simulink model "ddc_bpm_476_066"  (Simulink 7.8)
settings: Solver=ode45  StartTime=0.0  StopTime=2e-3  RelTol=1e-3
undefined symbols (not defined in the file): decim_factor_poly_35, dt_sim, frev_476, Fs_adc, n_ch, n_ovs, R_fofb, R_sec, R_sec_cfir, R_sec_pfir, xlipgetpartsetting
libraries: xbsIndex_r4 x1436, simulink x7
(part 3 of 12)

== system ddc_bpm_476_066/ST3 ==
  In : Inport
  Display : Display
  Sample Time : xbsIndex_r4/Sample Time  block_type=sampletime
      settings: infoedit="The Sample Time block reports the normalized sample period of its input.  A signal's normalized sample period is not equivalent to its Simulink absolute sample period.<br><br>Hardware notes: This block is implemented as a constant in hardware."
  out : xbsIndex_r4/Gateway Out  inherit_from_input=on  hdl_port=off  timing_constraint=Data Rate  locs_specified=off  LOCs={}  UseAsDAC=off  DACChannel='1'  block_type=gatewayout
      settings: infoedit="Gateway out block.  Converts Xilinx fixed-point or floating-point type inputs into ouputs of type Simulink integer, single, double, or fixed point.<br><br>Hardware notes:  In hardware these blocks become top level output ports or are discarded, depending on how they are configured."
  wires:
  out/1 -> Display/1
  Sample Time/1 -> out/1
  In/1 -> Sample Time/1

== system ddc_bpm_476_066/ST4 ==
  In : Inport
  Display : Display
  Sample Time : xbsIndex_r4/Sample Time  block_type=sampletime
      settings: infoedit="The Sample Time block reports the normalized sample period of its input.  A signal's normalized sample period is not equivalent to its Simulink absolute sample period.<br><br>Hardware notes: This block is implemented as a constant in hardware."
  out : xbsIndex_r4/Gateway Out  inherit_from_input=on  hdl_port=off  timing_constraint=Data Rate  locs_specified=off  LOCs={}  UseAsDAC=off  DACChannel='1'  block_type=gatewayout
      settings: infoedit="Gateway out block.  Converts Xilinx fixed-point or floating-point type inputs into ouputs of type Simulink integer, single, double, or fixed point.<br><br>Hardware notes:  In hardware these blocks become top level output ports or are discarded, depending on how they are configured."
  wires:
  out/1 -> Display/1
  Sample Time/1 -> out/1
  In/1 -> Sample Time/1

== system ddc_bpm_476_066/ST5 ==
  In : Inport
  Display : Display
  Sample Time : xbsIndex_r4/Sample Time  block_type=sampletime
      settings: infoedit="The Sample Time block reports the normalized sample period of its input.  A signal's normalized sample period is not equivalent to its Simulink absolute sample period.<br><br>Hardware notes: This block is implemented as a constant in hardware."
  out : xbsIndex_r4/Gateway Out  inherit_from_input=on  hdl_port=off  timing_constraint=Data Rate  locs_specified=off  LOCs={}  UseAsDAC=off  DACChannel='1'  block_type=gatewayout
      settings: infoedit="Gateway out block.  Converts Xilinx fixed-point or floating-point type inputs into ouputs of type Simulink integer, single, double, or fixed point.<br><br>Hardware notes:  In hardware these blocks become top level output ports or are discarded, depending on how they are configured."
  wires:
  out/1 -> Display/1
  Sample Time/1 -> out/1
  In/1 -> Sample Time/1

== system ddc_bpm_476_066/ST6 ==
  In : Inport
  Display : Display
  Sample Time : xbsIndex_r4/Sample Time  block_type=sampletime
      settings: infoedit="The Sample Time block reports the normalized sample period of its input.  A signal's normalized sample period is not equivalent to its Simulink absolute sample period.<br><br>Hardware notes: This block is implemented as a constant in hardware."
  out : xbsIndex_r4/Gateway Out  inherit_from_input=on  hdl_port=off  timing_constraint=Data Rate  locs_specified=off  LOCs={}  UseAsDAC=off  DACChannel='1'  block_type=gatewayout
      settings: infoedit="Gateway out block.  Converts Xilinx fixed-point or floating-point type inputs into ouputs of type Simulink integer, single, double, or fixed point.<br><br>Hardware notes:  In hardware these blocks become top level output ports or are discarded, depending on how they are configured."
  wires:
  out/1 -> Display/1
  Sample Time/1 -> out/1
  In/1 -> Sample Time/1

== system ddc_bpm_476_066/ST7 ==
  In : Inport
  Display : Display
  Sample Time : xbsIndex_r4/Sample Time  block_type=sampletime
      settings: infoedit="The Sample Time block reports the normalized sample period of its input.  A signal's normalized sample period is not equivalent to its Simulink absolute sample period.<br><br>Hardware notes: This block is implemented as a constant in hardware."
  out : xbsIndex_r4/Gateway Out  inherit_from_input=on  hdl_port=off  timing_constraint=Data Rate  locs_specified=off  LOCs={}  UseAsDAC=off  DACChannel='1'  block_type=gatewayout
      settings: infoedit="Gateway out block.  Converts Xilinx fixed-point or floating-point type inputs into ouputs of type Simulink integer, single, double, or fixed point.<br><br>Hardware notes:  In hardware these blocks become top level output ports or are discarded, depending on how they are configured."
  wires:
  out/1 -> Display/1
  Sample Time/1 -> out/1
  In/1 -> Sample Time/1

== system ddc_bpm_476_066/ST8 ==
  In : Inport
  Display : Display
  Sample Time : xbsIndex_r4/Sample Time  block_type=sampletime
      settings: infoedit="The Sample Time block reports the normalized sample period of its input.  A signal's normalized sample period is not equivalent to its Simulink absolute sample period.<br><br>Hardware notes: This block is implemented as a constant in hardware."
  X_monit1 : xbsIndex_r4/Gateway Out  inherit_from_input=on  hdl_port=off  timing_constraint=Data Rate  locs_specified=off  LOCs={}  UseAsDAC=off  DACChannel='1'  block_type=gatewayout
      settings: infoedit="Gateway out block.  Converts Xilinx fixed-point or floating-point type inputs into ouputs of type Simulink integer, single, double, or fixed point.<br><br>Hardware notes:  In hardware these blocks become top level output ports or are discarded, depending on how they are configured."
  wires:
  X_monit1/1 -> Display/1
  Sample Time/1 -> X_monit1/1
  In/1 -> Sample Time/1

== system ddc_bpm_476_066/ST9 ==
  In : Inport
  Display : Display
  Sample Time : xbsIndex_r4/Sample Time  block_type=sampletime
      settings: infoedit="The Sample Time block reports the normalized sample period of its input.  A signal's normalized sample period is not equivalent to its Simulink absolute sample period.<br><br>Hardware notes: This block is implemented as a constant in hardware."
  out : xbsIndex_r4/Gateway Out  inherit_from_input=on  hdl_port=off  timing_constraint=Data Rate  locs_specified=off  LOCs={}  UseAsDAC=off  DACChannel='1'  block_type=gatewayout
      settings: infoedit="Gateway out block.  Converts Xilinx fixed-point or floating-point type inputs into ouputs of type Simulink integer, single, double, or fixed point.<br><br>Hardware notes:  In hardware these blocks become top level output ports or are discarded, depending on how they are configured."
  wires:
  out/1 -> Display/1
  Sample Time/1 -> out/1
  In/1 -> Sample Time/1

== system ddc_bpm_476_066/TBT_amp ==
  Q_in0 : Inport
  I_in0 : Inport  Port=2
  ch_in0 : Inport  Port=3
  Q_in1 : Inport  Port=4
  I_in1 : Inport  Port=5
  ch_in1 : Inport  Port=6
  ST5 : Subsystem
  TBT_amp0 : Subsystem
  TBT_amp1 : Subsystem
  TDDM_tbt_amp_4ch : Subsystem
  Terminator{,1,3..4} (4 alike) : Terminator
  amp_out0 : Outport
  amp_out1 : Outport  Port=2
  amp_out2 : Outport  Port=3
  amp_out3 : Outport  Port=4
  wires:
  Q_in0/1 -> TBT_amp0/1(Q_in)
  I_in0/1 -> TBT_amp0/2(I_in)
  ch_in0/1 -> TBT_amp0/3(ch_in)
  Q_in1/1 -> TBT_amp1/1(Q_in)
  I_in1/1 -> TBT_amp1/2(I_in)
  ch_in1/1 -> TBT_amp1/3(ch_in)
  TBT_amp0/2(phase_out) -> Terminator/1
  TBT_amp0/3(valid_out) -> Terminator1/1
  TBT_amp1/2(phase_out) -> Terminator3/1
  TBT_amp1/3(valid_out) -> Terminator4/1
  TBT_amp0/1(amp_out) -> TDDM_tbt_amp_4ch/1(amp_in0), ST5/1(In)
  TBT_amp0/4(ch_out) -> TDDM_tbt_amp_4ch/2(ch_in0)
  TBT_amp1/1(amp_out) -> TDDM_tbt_amp_4ch/3(amp_in1)
  TBT_amp1/4(ch_out) -> TDDM_tbt_amp_4ch/4(ch_in1)
  TDDM_tbt_amp_4ch/1(amp_out0) -> amp_out0/1
  TDDM_tbt_amp_4ch/2(amp_out1) -> amp_out1/1
  TDDM_tbt_amp_4ch/3(amp_out2) -> amp_out2/1
  TDDM_tbt_amp_4ch/4(amp_out3) -> amp_out3/1

== system ddc_bpm_476_066/TDM_mix ==
  din_ch0 : Inport
  din_ch1 : Inport  Port=2
  din_ch2 : Inport  Port=3
  din_ch3 : Inport  Port=4
  Constant10 : xbsIndex_r4/Constant  const=0  gui_display_data_type=Boolean  arith_type=Boolean  n_bits=16  bin_pt=14  preci_type=Single  exp_width=8  frac_width=24  explicit_period=on  period=1/Fs_adc/n_ovs  equ=P=C  opselect=C  inp2=PCIN>>17  opr=+  inp1=P  carry=CIN  dbl_ovrd=off  block_type=constant
  Constant11 : xbsIndex_r4/Constant  const=0  gui_display_data_type=Boolean  arith_type=Boolean  n_bits=16  bin_pt=14  preci_type=Single  exp_width=8  frac_width=24  explicit_period=on  period=1/Fs_adc/n_ovs  equ=P=C  opselect=C  inp2=PCIN>>17  opr=+  inp1=P  carry=CIN  dbl_ovrd=off  block_type=constant
  ST1 : Subsystem
  ST2 : Subsystem
  ST3 : Subsystem
  ST4 : Subsystem
  ST5 : Subsystem
  ST6 : Subsystem
  TDM_mix_ch0_1 : Subsystem
  TDM_mix_ch0_2 : Subsystem
  dout0 : Outport
  ch_out0 : Outport  Port=2
  dout1 : Outport  Port=3
  ch_out1 : Outport  Port=4
  wires:
  Constant10/1 -> TDM_mix_ch0_1/1(rst), ST3/1(In)
  Constant11/1 -> ST5/1(In), TDM_mix_ch0_2/1(rst)
  TDM_mix_ch0_1/1(dout) -> dout0/1, ST1/1(In)
  din_ch0/1 -> TDM_mix_ch0_1/2(din_ch0)
  TDM_mix_ch0_1/2(ch_out) -> ch_out0/1
  din_ch1/1 -> TDM_mix_ch0_1/3(din_ch1), ST2/1(In)
  TDM_mix_ch0_2/1(dout) -> dout1/1, ST4/1(In)
  din_ch2/1 -> TDM_mix_ch0_2/2(din_ch0)
  TDM_mix_ch0_2/2(ch_out) -> ch_out1/1
  din_ch3/1 -> ST6/1(In), TDM_mix_ch0_2/3(din_ch1)

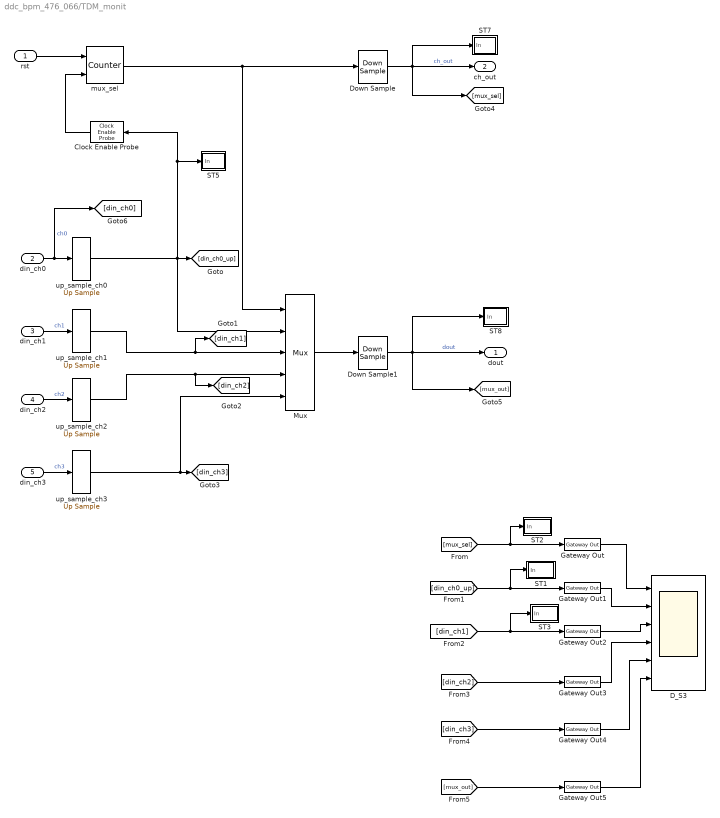
== system ddc_bpm_476_066/TDM_monit ==
  rst : Inport
  din_ch0 : Inport  Port=2
  din_ch1 : Inport  Port=3
  din_ch2 : Inport  Port=4
  din_ch3 : Inport  Port=5
  Clock Enable Probe : xbsIndex_r4/Clock Enable Probe  inherit_constraints=on  block_type=ceprobe
      settings: infoedit="Clock enable extractor.  Produces a Boolean output that mirrors the hardware clock enable associated with the input sample rate.<br><br>Hardware notes: in hardware this block costs nothing."
  D_S3 : Scope  NumInputPorts=6
      settings: TimeRange=0.0004  YMin=-1~-1.5~10~-1.5~-5~-5  YMax=1~1.5~100~1.5~5~5  MaxDataPoints=1000000  SampleInput=on
  Down Sample : xbsIndex_r4/Down Sample  sample_ratio=R_fofb*n_ovs/n_ch  sample_phase="Last Value of Frame  (most efficient)"  en=off  latency=1  dbl_ovrd=off  block_type=dsamp
  Down Sample1 : xbsIndex_r4/Down Sample  sample_ratio=R_fofb*n_ovs/n_ch  sample_phase="Last Value of Frame  (most efficient)"  en=off  latency=1  dbl_ovrd=off  block_type=dsamp
  Gateway Out{,1..5} (6 alike) : xbsIndex_r4/Gateway Out  inherit_from_input=on  hdl_port=off  timing_constraint=None  locs_specified=off  LOCs={}  UseAsDAC=off  DACChannel='1'  block_type=gatewayout
      settings: infoedit="Gateway out block.  Converts Xilinx fixed-point or floating-point type inputs into ouputs of type Simulink integer, single, double, or fixed point.<br><br>Hardware notes:  In hardware these blocks become top level output ports or are discarded, depending on how they are configured."
  Mux : xbsIndex_r4/Mux  inputs=4  en=off  latency=0  precision=Full  arith_type=Unsigned  n_bits=16  bin_pt=14  quantization=Truncate  overflow=Wrap  dbl_ovrd=off  block_type=mux
  ST1 : Subsystem
  ST2 : Subsystem
  ST3 : Subsystem
  ST5 : Subsystem
  ST7 : Subsystem
  ST8 : Subsystem
  mux_sel : xbsIndex_r4/Counter  cnt_type=Free Running  cnt_to=Inf  operation=Up  start_count=0  cnt_by_val=1  arith_type=Unsigned  n_bits=2  bin_pt=0  load_pin=off  rst=on  en=on  explicit_period=off  period=1/Fs_adc/4*1112  dbl_ovrd=off  use_behavioral_HDL=off  implementation=Fabric  block_type=counter
  up_sample_ch{0..3} (4 alike) : xbsIndex_r4/Up Sample  sample_ratio=n_ch  copy_samples=on  en=off  latency=0  dbl_ovrd=off  block_type=usamp
  dout : Outport
  ch_out : Outport  Port=2
  wires:
  Mux/1 -> Down Sample1/1
  mux_sel/1 -> Mux/1, Down Sample/1
  up_sample_ch3/1 -> Mux/5, [din_ch3]
  up_sample_ch2/1 -> Mux/4, [din_ch2]
  up_sample_ch1/1 -> Mux/3, [din_ch1]
  up_sample_ch0/1 -> Mux/2, [din_ch0_up], Clock Enable Probe/1, ST5/1(In)
  din_ch0/1 -> [din_ch0], up_sample_ch0/1  "ch0"
  din_ch1/1 -> up_sample_ch1/1  "ch1"
  Down Sample1/1 -> dout/1, [mux_out], ST8/1(In)  "dout"
  din_ch2/1 -> up_sample_ch2/1  "ch2"
  din_ch3/1 -> up_sample_ch3/1  "ch3"
  Down Sample/1 -> ch_out/1, [mux_sel], ST7/1(In)  "ch_out"
  Gateway Out/1 -> D_S3/1
  Gateway Out1/1 -> D_S3/2
  Gateway Out4/1 -> D_S3/5
  Gateway Out3/1 -> D_S3/4
  Gateway Out2/1 -> D_S3/3
  [mux_sel] -> Gateway Out/1, ST2/1(In)
  [din_ch0_up] -> Gateway Out1/1, ST1/1(In)
  [din_ch1] -> Gateway Out2/1, ST3/1(In)
  [din_ch3] -> Gateway Out4/1
  [din_ch2] -> Gateway Out3/1
  [mux_out] -> Gateway Out5/1
  Gateway Out5/1 -> D_S3/6
  Clock Enable Probe/1 -> mux_sel/2
  rst/1 -> mux_sel/1

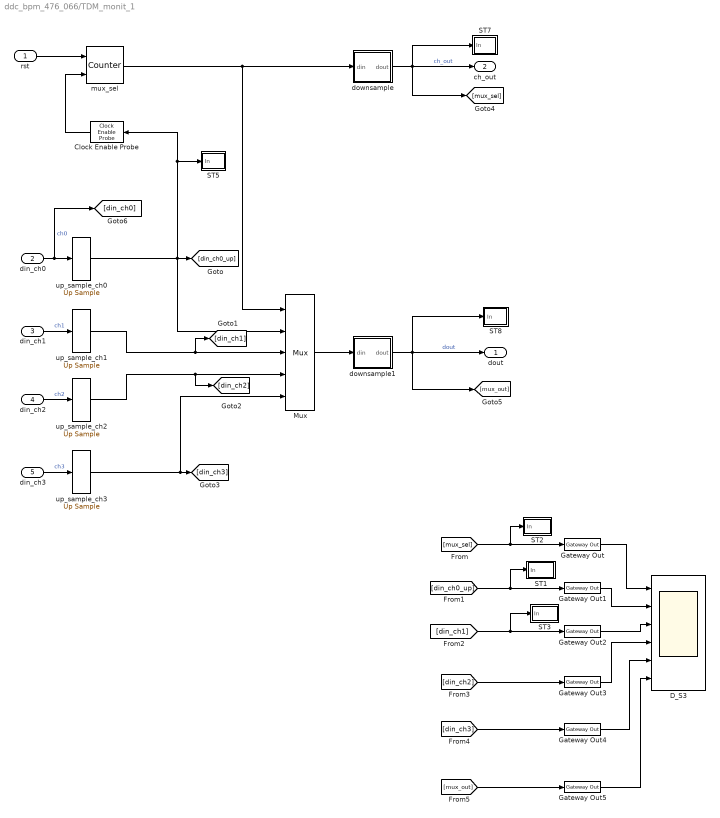
== system ddc_bpm_476_066/TDM_monit_1 ==
  rst : Inport
  din_ch0 : Inport  Port=2
  din_ch1 : Inport  Port=3
  din_ch2 : Inport  Port=4
  din_ch3 : Inport  Port=5
  Clock Enable Probe : xbsIndex_r4/Clock Enable Probe  inherit_constraints=on  block_type=ceprobe
      settings: infoedit="Clock enable extractor.  Produces a Boolean output that mirrors the hardware clock enable associated with the input sample rate.<br><br>Hardware notes: in hardware this block costs nothing."
  D_S3 : Scope  NumInputPorts=6
      settings: TimeRange=0.0004  YMin=-1~-1.5~10~-1.5~-5~-5  YMax=1~1.5~100~1.5~5~5  MaxDataPoints=1000000  SampleInput=on
  Gateway Out{,1..5} (6 alike) : xbsIndex_r4/Gateway Out  inherit_from_input=on  hdl_port=off  timing_constraint=None  locs_specified=off  LOCs={}  UseAsDAC=off  DACChannel='1'  block_type=gatewayout
      settings: infoedit="Gateway out block.  Converts Xilinx fixed-point or floating-point type inputs into ouputs of type Simulink integer, single, double, or fixed point.<br><br>Hardware notes:  In hardware these blocks become top level output ports or are discarded, depending on how they are configured."
  Mux : xbsIndex_r4/Mux  inputs=4  en=off  latency=0  precision=Full  arith_type=Unsigned  n_bits=16  bin_pt=14  quantization=Truncate  overflow=Wrap  dbl_ovrd=off  block_type=mux
  ST1 : Subsystem
  ST2 : Subsystem
  ST3 : Subsystem
  ST5 : Subsystem
  ST7 : Subsystem
  ST8 : Subsystem
  downsample : Subsystem
  downsample1 : Subsystem
  mux_sel : xbsIndex_r4/Counter  cnt_type=Free Running  cnt_to=Inf  operation=Up  start_count=0  cnt_by_val=1  arith_type=Unsigned  n_bits=2  bin_pt=0  load_pin=off  rst=on  en=on  explicit_period=off  period=1/Fs_adc/4*1112  dbl_ovrd=off  use_behavioral_HDL=off  implementation=Fabric  block_type=counter
  up_sample_ch{0..3} (4 alike) : xbsIndex_r4/Up Sample  sample_ratio=n_ch  copy_samples=on  en=off  latency=0  dbl_ovrd=off  block_type=usamp
  dout : Outport
  ch_out : Outport  Port=2
  wires:
  Mux/1 -> downsample1/1(din)
  mux_sel/1 -> Mux/1, downsample/1(din)
  up_sample_ch3/1 -> Mux/5, [din_ch3]
  up_sample_ch2/1 -> Mux/4, [din_ch2]
  up_sample_ch1/1 -> Mux/3, [din_ch1]
  up_sample_ch0/1 -> Mux/2, [din_ch0_up], Clock Enable Probe/1, ST5/1(In)
  din_ch0/1 -> [din_ch0], up_sample_ch0/1  "ch0"
  din_ch1/1 -> up_sample_ch1/1  "ch1"
  downsample1/1(dout) -> dout/1, [mux_out], ST8/1(In)  "dout"
  din_ch2/1 -> up_sample_ch2/1  "ch2"
  din_ch3/1 -> up_sample_ch3/1  "ch3"
  downsample/1(dout) -> ch_out/1, [mux_sel], ST7/1(In)  "ch_out"
  Gateway Out/1 -> D_S3/1
  Gateway Out1/1 -> D_S3/2
  Gateway Out4/1 -> D_S3/5
  Gateway Out3/1 -> D_S3/4
  Gateway Out2/1 -> D_S3/3
  [mux_sel] -> Gateway Out/1, ST2/1(In)
  [din_ch0_up] -> Gateway Out1/1, ST1/1(In)
  [din_ch1] -> Gateway Out2/1, ST3/1(In)
  [din_ch3] -> Gateway Out4/1
  [din_ch2] -> Gateway Out3/1
  [mux_out] -> Gateway Out5/1
  Gateway Out5/1 -> D_S3/6
  Clock Enable Probe/1 -> mux_sel/2
  rst/1 -> mux_sel/1

== system ddc_bpm_476_066/debug_analysis ==
  Constant{,1..3} (4 alike) : Constant  Value=0
  D_S2 : Scope  NumInputPorts=2
      settings: TimeRange=0.0004  YMin=1~1  YMax=1~1  SaveName=ScopeData8  MaxDataPoints=1000000  SampleInput=on
  D_S3 : Scope  NumInputPorts=4
      settings: TimeRange=0.0004  YMin=-1~-1.5~10~-1.5  YMax=1~1.5~100~1.5  SaveName=ScopeData9  MaxDataPoints=1000000  SampleInput=on
  D_S4 : Scope  NumInputPorts=4
      settings: TimeRange=0.0004  YMin=0.95~0~10~-1.5  YMax=1.05~60~100~1.5  SaveName=ScopeData10  MaxDataPoints=1000000  SampleInput=on
  q_tbt_o3 : xbsIndex_r4/Gateway Out  inherit_from_input=on  hdl_port=off  timing_constraint=None  locs_specified=off  LOCs={}  UseAsDAC=off  DACChannel='1'  block_type=gatewayout
      settings: infoedit="Gateway out block.  Converts Xilinx fixed-point or floating-point type inputs into ouputs of type Simulink integer, single, double, or fixed point.<br><br>Hardware notes:  In hardware these blocks become top level output ports or are discarded, depending on how they are configured."
  sum_tbt_o3 : xbsIndex_r4/Gateway Out  inherit_from_input=on  hdl_port=off  timing_constraint=None  locs_specified=off  LOCs={}  UseAsDAC=off  DACChannel='1'  block_type=gatewayout
      settings: infoedit="Gateway out block.  Converts Xilinx fixed-point or floating-point type inputs into ouputs of type Simulink integer, single, double, or fixed point.<br><br>Hardware notes:  In hardware these blocks become top level output ports or are discarded, depending on how they are configured."
  x_tbt_o3 : xbsIndex_r4/Gateway Out  inherit_from_input=on  hdl_port=off  timing_constraint=None  locs_specified=off  LOCs={}  UseAsDAC=off  DACChannel='1'  block_type=gatewayout
      settings: infoedit="Gateway out block.  Converts Xilinx fixed-point or floating-point type inputs into ouputs of type Simulink integer, single, double, or fixed point.<br><br>Hardware notes:  In hardware these blocks become top level output ports or are discarded, depending on how they are configured."
  x_tbt_o4 : xbsIndex_r4/Gateway Out  inherit_from_input=on  hdl_port=off  timing_constraint=None  locs_specified=off  LOCs={}  UseAsDAC=off  DACChannel='1'  block_type=gatewayout
      settings: infoedit="Gateway out block.  Converts Xilinx fixed-point or floating-point type inputs into ouputs of type Simulink integer, single, double, or fixed point.<br><br>Hardware notes:  In hardware these blocks become top level output ports or are discarded, depending on how they are configured."
  y_tbt_o4 : xbsIndex_r4/Gateway Out  inherit_from_input=on  hdl_port=off  timing_constraint=None  locs_specified=off  LOCs={}  UseAsDAC=off  DACChannel='1'  block_type=gatewayout
      settings: infoedit="Gateway out block.  Converts Xilinx fixed-point or floating-point type inputs into ouputs of type Simulink integer, single, double, or fixed point.<br><br>Hardware notes:  In hardware these blocks become top level output ports or are discarded, depending on how they are configured."
  y_tbt_o7 : xbsIndex_r4/Gateway Out  inherit_from_input=on  hdl_port=off  timing_constraint=None  locs_specified=off  LOCs={}  UseAsDAC=off  DACChannel='1'  block_type=gatewayout
      settings: infoedit="Gateway out block.  Converts Xilinx fixed-point or floating-point type inputs into ouputs of type Simulink integer, single, double, or fixed point.<br><br>Hardware notes:  In hardware these blocks become top level output ports or are discarded, depending on how they are configured."
  wires:
  [Y_DIVIDEND_D_S_FPGA_RDY] -> q_tbt_o3/1
  [Y_DIVIDEND_D_S_FPGA] -> x_tbt_o3/1
  x_tbt_o3/1 -> D_S3/1
  [SUM_DIVISOR_D_S_FPGA] -> x_tbt_o4/1
  [SUM_DIVISOR_D_S_FPGA_VALID] -> y_tbt_o4/1
  x_tbt_o4/1 -> D_S3/3
  y_tbt_o4/1 -> D_S3/4
  [D_S_FPGA_Y_DIVIDER_QUOC] -> y_tbt_o7/1
  y_tbt_o7/1 -> D_S4/3
  Constant/1 -> D_S4/4
  q_tbt_o3/1 -> D_S2/1
  Constant1/1 -> D_S4/1
  Constant2/1 -> D_S4/2
  Constant3/1 -> D_S3/2
  [Y_DIVIDOR_D_S_FPGA_RDY] -> sum_tbt_o3/1
  sum_tbt_o3/1 -> D_S2/2

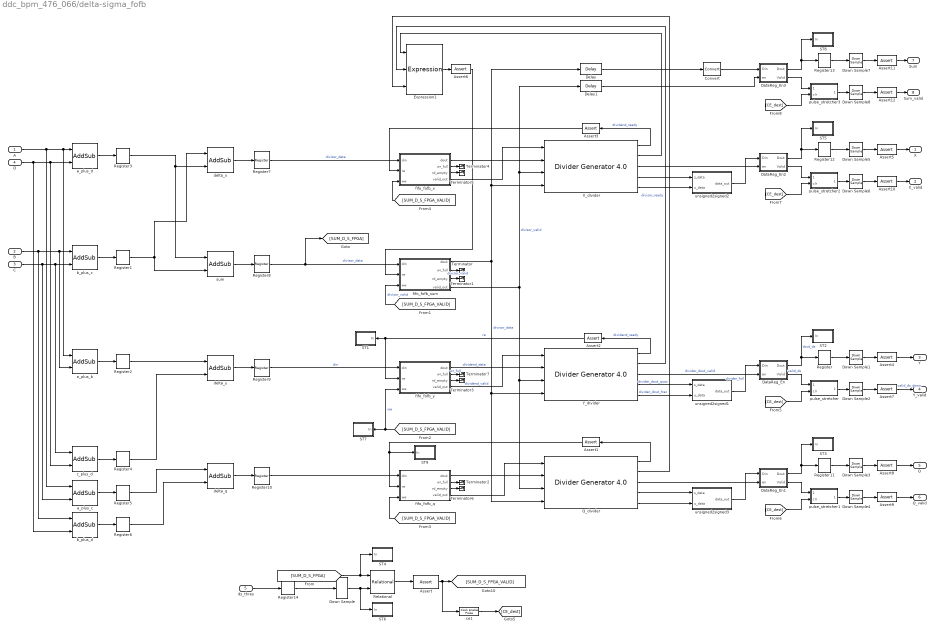
== system ddc_bpm_476_066/delta-sigma_fofb ==
  A : Inport
  B : Inport  Port=2
  C : Inport  Port=3
  D : Inport  Port=4
  ds_thres : Inport  Port=5
  Assert : xbsIndex_r4/Assert  assert_type=off  type_source=Explicitly  gui_display_data_type=Fixed-point  arith_type="Signed  (2's comp)"  n_bits=16  bin_pt=14  preci_type=Single  exp_width=8  frac_width=24  assert_rate=on  rate_source=Explicitly  period=(1/Fs_adc/n_ovs)*(R_fofb*n_ovs)  output_port=on  block_type=assert
  Assert{1..3,6} (4 alike) : xbsIndex_r4/Assert  assert_type=off  type_source=Explicitly  gui_display_data_type=Fixed-point  arith_type="Signed  (2's comp)"  n_bits=16  bin_pt=14  preci_type=Single  exp_width=8  frac_width=24  assert_rate=on  rate_source=Explicitly  period=1/Fs_adc/n_ovs  output_port=on  block_type=assert
  Assert{4..5,7..12} (8 alike) : xbsIndex_r4/Assert  assert_type=off  type_source=Explicitly  gui_display_data_type=Fixed-point  arith_type="Signed  (2's comp)"  n_bits=16  bin_pt=14  preci_type=Single  exp_width=8  frac_width=24  assert_rate=on  rate_source=Explicitly  period=(1/Fs_adc/n_ovs)*R_fofb*n_ovs  output_port=on  block_type=assert
  Convert : xbsIndex_r4/Convert  gui_display_data_type=Fixed-point  arith_type="Signed  (2's comp)"  n_bits=25  bin_pt=21  float_type=Single  exp_bits=8  fraction_bits=24  quantization="Round  (unbiased: +/- Inf)"  overflow=Saturate  en=off  latency=0  dbl_ovrd=off  pipeline=off  block_type=convert
  DataReg_En : Subsystem
  DataReg_En1 : Subsystem
  DataReg_En2 : Subsystem
  DataReg_En3 : Subsystem
  Delay : xbsIndex_r4/Delay  rst=off  infoeditControl=Selection of Reset will increase slice count due to use of real FFs and instead of SRLs  en=off  latency=25  dbl_ovrd=off  reg_retiming=off  block_type=delay
  Delay1 : xbsIndex_r4/Delay  rst=off  infoeditControl=Selection of Reset will increase slice count due to use of real FFs and instead of SRLs  en=off  latency=25  dbl_ovrd=off  reg_retiming=off  block_type=delay
  Down Sample : xbsIndex_r4/Down Sample  sample_ratio=R_fofb  sample_phase="Last Value of Frame  (most efficient)"  en=off  latency=1  dbl_ovrd=off  block_type=dsamp
  Down Sample{1..8} (8 alike) : xbsIndex_r4/Down Sample  sample_ratio=R_fofb*n_ovs  sample_phase="Last Value of Frame  (most efficient)"  en=off  latency=1  dbl_ovrd=off  block_type=dsamp
  Expression1 : xbsIndex_r4/Expression  expression=a & b & c  align_bp=on  en=off  latency=0  precision=Full  arith_type=Unsigned  n_bits=16  bin_pt=0  dbl_ovrd=off  block_type=expr
  Q_divider : xbsIndex_r4/Divider Generator 4.0   algorithm_type=High_Radix  remainder_type=Fractional  fractional_width=24  clocks_per_division=1  divide_by_zero_detect=off  flowcontrol=NonBlocking  optimizegoal=Performance  latency_configuration=Manual  latency=25  dividend_has_tuser=off  dividend_has_tlast=off  divisor_has_tuser=off  divisor_has_tlast=off  aclken=off  aresetn=off  outtready=off  outtlastbehv=Null  trim_axipin_name=on  dividend_tuser_width=1  divisor_tuser_width=1  operand_sign=Signed  dividend_and_quotient_width=16  divisor_width=16  ip_name=Divider Generator  ip_version=4.0  dsptool_ready=true  ipcore_usecache=true  ipcore_useipmodelcache=true  wrapper_available=true  port_translation_map={'aclken' => 'en','aresetn' => 'rst'}  ipcore_fpga_part=xlipgetpartsetting(gcb, {'virtex7', 'xc7v1500t', '-2', 'fhg1157'})  ipcore_verbose=false  block_type=div_gen_v4_0
      settings: infoedit=Divider Generator 4.0
  Register{,1..14} (15 alike) : xbsIndex_r4/Register  init=0  rst=off  en=off  dbl_ovrd=off  block_type=register
  Relational : xbsIndex_r4/Relational  mode=a>b  en=off  latency=1  dbl_ovrd=off  block_type=relational
  ST1 : Subsystem
  ST2 : Subsystem
  ST3 : Subsystem
  ST4 : Subsystem
  ST5 : Subsystem
  ST6 : Subsystem
  ST7 : Subsystem
  ST8 : Subsystem
  ST9 : Subsystem
  Terminator{,1..7} (8 alike) : Terminator
  X_divider : xbsIndex_r4/Divider Generator 4.0   algorithm_type=High_Radix  remainder_type=Fractional  fractional_width=24  clocks_per_division=1  divide_by_zero_detect=off  flowcontrol=NonBlocking  optimizegoal=Performance  latency_configuration=Manual  latency=25  dividend_has_tuser=off  dividend_has_tlast=off  divisor_has_tuser=off  divisor_has_tlast=off  aclken=off  aresetn=off  outtready=off  outtlastbehv=Null  trim_axipin_name=on  dividend_tuser_width=1  divisor_tuser_width=1  operand_sign=Signed  dividend_and_quotient_width=16  divisor_width=16  ip_name=Divider Generator  ip_version=4.0  dsptool_ready=true  ipcore_usecache=true  ipcore_useipmodelcache=true  wrapper_available=true  port_translation_map={'aclken' => 'en','aresetn' => 'rst'}  ipcore_fpga_part=xlipgetpartsetting(gcb, {'virtex7', 'xc7v1500t', '-2', 'fhg1157'})  ipcore_verbose=false  block_type=div_gen_v4_0
      settings: infoedit=Divider Generator 4.0
  Y_divider : xbsIndex_r4/Divider Generator 4.0   algorithm_type=High_Radix  remainder_type=Fractional  fractional_width=24  clocks_per_division=1  divide_by_zero_detect=off  flowcontrol=NonBlocking  optimizegoal=Performance  latency_configuration=Manual  latency=25  dividend_has_tuser=off  dividend_has_tlast=off  divisor_has_tuser=off  divisor_has_tlast=off  aclken=off  aresetn=off  outtready=off  outtlastbehv=Null  trim_axipin_name=on  dividend_tuser_width=1  divisor_tuser_width=1  operand_sign=Signed  dividend_and_quotient_width=16  divisor_width=16  ip_name=Divider Generator  ip_version=4.0  dsptool_ready=true  ipcore_usecache=true  ipcore_useipmodelcache=true  wrapper_available=true  port_translation_map={'aclken' => 'en','aresetn' => 'rst'}  ipcore_fpga_part=xlipgetpartsetting(gcb, {'virtex7', 'xc7v1500t', '-2', 'fhg1157'})  ipcore_verbose=false  block_type=div_gen_v4_0
      settings: infoedit=Divider Generator 4.0
  a_plus_b : xbsIndex_r4/AddSub  mode=Addition  use_carryin=off  use_carryout=off  en=off  latency=0  precision=Full  arith_type=Unsigned  n_bits=16  bin_pt=14  quantization=Truncate  overflow=Wrap  dbl_ovrd=off  use_behavioral_HDL=off  hw_selection=Fabric  pipelined=off  block_type=addsub
  a_plus_c : xbsIndex_r4/AddSub  mode=Addition  use_carryin=off  use_carryout=off  en=off  latency=0  precision=Full  arith_type=Unsigned  n_bits=16  bin_pt=14  quantization=Truncate  overflow=Wrap  dbl_ovrd=off  use_behavioral_HDL=off  hw_selection=Fabric  pipelined=off  block_type=addsub
  a_plus_d : xbsIndex_r4/AddSub  mode=Addition  use_carryin=off  use_carryout=off  en=off  latency=0  precision=Full  arith_type=Unsigned  n_bits=16  bin_pt=14  quantization=Truncate  overflow=Wrap  dbl_ovrd=off  use_behavioral_HDL=off  hw_selection=Fabric  pipelined=off  block_type=addsub
  b_plus_c : xbsIndex_r4/AddSub  mode=Addition  use_carryin=off  use_carryout=off  en=off  latency=0  precision=Full  arith_type=Unsigned  n_bits=16  bin_pt=14  quantization=Truncate  overflow=Wrap  dbl_ovrd=off  use_behavioral_HDL=off  hw_selection=Fabric  pipelined=off  block_type=addsub
  b_plus_d : xbsIndex_r4/AddSub  mode=Addition  use_carryin=off  use_carryout=off  en=off  latency=0  precision=Full  arith_type=Unsigned  n_bits=16  bin_pt=14  quantization=Truncate  overflow=Wrap  dbl_ovrd=off  use_behavioral_HDL=off  hw_selection=Fabric  pipelined=off  block_type=addsub
  c_plus_d : xbsIndex_r4/AddSub  mode=Addition  use_carryin=off  use_carryout=off  en=off  latency=0  precision=Full  arith_type=Unsigned  n_bits=16  bin_pt=14  quantization=Truncate  overflow=Wrap  dbl_ovrd=off  use_behavioral_HDL=off  hw_selection=Fabric  pipelined=off  block_type=addsub
  ce1 : xbsIndex_r4/Clock Enable Probe  inherit_constraints=on  block_type=ceprobe
      settings: infoedit="Clock enable extractor.  Produces a Boolean output that mirrors the hardware clock enable associated with the input sample rate.<br><br>Hardware notes: in hardware this block costs nothing."
  delta_q : xbsIndex_r4/AddSub  mode=Subtraction  use_carryin=off  use_carryout=off  en=off  latency=0  precision=Full  arith_type=Unsigned  n_bits=16  bin_pt=14  quantization=Truncate  overflow=Wrap  dbl_ovrd=off  use_behavioral_HDL=off  hw_selection=Fabric  pipelined=off  block_type=addsub
  delta_x : xbsIndex_r4/AddSub  mode=Subtraction  use_carryin=off  use_carryout=off  en=off  latency=0  precision=Full  arith_type=Unsigned  n_bits=16  bin_pt=14  quantization=Truncate  overflow=Wrap  dbl_ovrd=off  use_behavioral_HDL=off  hw_selection=Fabric  pipelined=off  block_type=addsub
  delta_y : xbsIndex_r4/AddSub  mode=Subtraction  use_carryin=off  use_carryout=off  en=off  latency=0  precision=Full  arith_type=Unsigned  n_bits=16  bin_pt=14  quantization=Truncate  overflow=Wrap  dbl_ovrd=off  use_behavioral_HDL=off  hw_selection=Fabric  pipelined=off  block_type=addsub
  fifo_fofb_q : Subsystem
  fifo_fofb_sum : Subsystem
  fifo_fofb_x : Subsystem
  fifo_fofb_y : Subsystem
  pulse_stretcher : Subsystem
  pulse_stretcher1 : Subsystem
  pulse_stretcher2 : Subsystem
  pulse_stretcher3 : Subsystem
  sum : xbsIndex_r4/AddSub  mode=Addition  use_carryin=off  use_carryout=off  en=off  latency=0  precision=Full  arith_type=Unsigned  n_bits=16  bin_pt=14  quantization=Truncate  overflow=Wrap  dbl_ovrd=off  use_behavioral_HDL=off  hw_selection=Fabric  pipelined=off  block_type=addsub
  unsigned2signed1 : Subsystem
  unsigned2signed2 : Subsystem
  unsigned2signed3 : Subsystem
  X : Outport
  X_valid : Outport  Port=2
  Y : Outport  Port=3
  Y_valid : Outport  Port=4
  Q : Outport  Port=5
  Q_valid : Outport  Port=6
  Sum : Outport  Port=7
  Sum_valid : Outport  Port=8
  wires:
  A/1 -> a_plus_d/1, a_plus_b/1, a_plus_c/1
  D/1 -> a_plus_d/2, c_plus_d/2, b_plus_d/2
  B/1 -> b_plus_c/1, a_plus_b/2, b_plus_d/1
  C/1 -> b_plus_c/2, c_plus_d/1, a_plus_c/2
  a_plus_d/1 -> Register3/1
  b_plus_c/1 -> Register1/1
  a_plus_b/1 -> Register2/1
  c_plus_d/1 -> Register4/1
  a_plus_c/1 -> Register5/1
  b_plus_d/1 -> Register6/1
  Register3/1 -> sum/1, delta_x/2
  Register1/1 -> sum/2, delta_x/1
  Register2/1 -> delta_y/1
  Register4/1 -> delta_y/2
  Register5/1 -> delta_q/1
  Register6/1 -> delta_q/2
  delta_q/1 -> Register10/1
  delta_x/1 -> Register7/1
  Register8/1 -> fifo_fofb_sum/1(din), [SUM_D_S_FPGA]  "divisor_data"
  sum/1 -> Register8/1
  delta_y/1 -> Register9/1
  Delay/1 -> Convert/1
  Register7/1 -> fifo_fofb_x/1(din)  "divisor_data"
  Y_divider/5 -> unsigned2signed1/2(u_data)  "divider_dout_frac"
  Y_divider/3 -> DataReg_En/2(en)  "divider_dout_valid"
  Register9/1 -> fifo_fofb_y/1(din)  "din"
  Register10/1 -> fifo_fofb_q/1(din)
  X_divider/2 -> Expression1/1
  Y_divider/2 -> Expression1/2  "divisor_ready"
  ds_thres/1 -> Register14/1
  [SUM_D_S_FPGA] -> Relational/1, ST4/1(In)
  Relational/1 -> Assert/1
  fifo_fofb_x/1(dout) -> X_divider/2
  fifo_fofb_q/1(dout) -> Q_divider/2
  Q_divider/2 -> Expression1/3
  Q_divider/1 -> Assert1/1
  fifo_fofb_q/4(valid_out) -> Q_divider/1
  fifo_fofb_x/4(valid_out) -> X_divider/1
  X_divider/5 -> unsigned2signed2/2(u_data)
  X_divider/4 -> unsigned2signed2/1(s_data)
  Y_divider/4 -> unsigned2signed1/1(s_data)  "divider_dout_quoc"
  unsigned2signed1/1(data_out) -> DataReg_En/1(Din)  "divider_full"
  Q_divider/5 -> unsigned2signed3/2(u_data)
  Q_divider/4 -> unsigned2signed3/1(s_data)
  Assert/1 -> ce1/1, [SUM_D_S_FPGA_VALID]
  Down Sample/1 -> ST6/1(In), Relational/2
  fifo_fofb_y/1(dout) -> Y_divider/2  "dividend_data"
  [SUM_D_S_FPGA_VALID] -> ST7/1(In), fifo_fofb_y/3(we)  "we"
  [SUM_D_S_FPGA_VALID] -> fifo_fofb_sum/3(we)  "divisor_valid"
  Expression1/1 -> Assert6/1
  [SUM_D_S_FPGA_VALID] -> fifo_fofb_x/3(we)
  [SUM_D_S_FPGA_VALID] -> fifo_fofb_q/3(we)
  fifo_fofb_y/4(valid_out) -> Y_divider/1  "dividend_valid"
  fifo_fofb_sum/4(valid_out) -> Q_divider/3, Y_divider/3, X_divider/3, Delay1/1  "divisor_valid"
  fifo_fofb_sum/2(wr_full) -> Terminator/1  "divisor_valid"
  fifo_fofb_sum/3(rd_empty) -> Terminator1/1
  fifo_fofb_x/2(wr_full) -> Terminator4/1
  fifo_fofb_x/3(rd_empty) -> Terminator5/1
  fifo_fofb_sum/1(dout) -> Q_divider/4, Y_divider/4, X_divider/4, Delay/1  "divisor_data"
  fifo_fofb_q/2(wr_full) -> Terminator2/1
  fifo_fofb_y/3(rd_empty) -> Terminator3/1
  Register14/1 -> Down Sample/1
  DataReg_En/1(Dout) -> ST2/1(In), Register/1  "dout_ds"
  fifo_fofb_q/3(rd_empty) -> Terminator6/1
  Assert7/1 -> Y_valid/1  "valid_ds_down"
  Assert4/1 -> Y/1
  Assert1/1 -> ST9/1(In), fifo_fofb_q/2(re)
  Assert2/1 -> ST1/1(In), fifo_fofb_y/2(re)  "re"
  Assert3/1 -> fifo_fofb_x/2(re)
  Assert6/1 -> fifo_fofb_sum/2(re)
  Y_divider/1 -> Assert2/1  "dividend_ready"
  X_divider/1 -> Assert3/1  "dividend_ready"
  DataReg_En/2(Valid) -> pulse_stretcher/1(pulse_in)  "valid_ds"
  pulse_stretcher/1(extd_out) -> Down Sample2/1
  Down Sample1/1 -> Assert4/1
  Down Sample2/1 -> Assert7/1
  Register/1 -> Down Sample1/1
  ce1/1 -> [CE_dest]
  [CE_dest] -> pulse_stretcher/2(clr)
  unsigned2signed3/1(data_out) -> DataReg_En1/1(Din)
  DataReg_En1/1(Dout) -> ST3/1(In), Register11/1
  Assert9/1 -> Q_valid/1
  Assert8/1 -> Q/1
  DataReg_En1/2(Valid) -> pulse_stretcher1/1(pulse_in)
  pulse_stretcher1/1(extd_out) -> Down Sample4/1
  Down Sample3/1 -> Assert8/1
  Down Sample4/1 -> Assert9/1
  Register11/1 -> Down Sample3/1
  [CE_dest] -> pulse_stretcher1/2(clr)
  Q_divider/3 -> DataReg_En1/2(en)
  unsigned2signed2/1(data_out) -> DataReg_En2/1(Din)
  DataReg_En2/1(Dout) -> ST5/1(In), Register12/1
  DataReg_En2/2(Valid) -> pulse_stretcher2/1(pulse_in)
  pulse_stretcher2/1(extd_out) -> Down Sample6/1
  Down Sample5/1 -> Assert5/1
  Down Sample6/1 -> Assert10/1
  Register12/1 -> Down Sample5/1
  [CE_dest] -> pulse_stretcher2/2(clr)
  X_divider/3 -> DataReg_En2/2(en)
  Assert5/1 -> X/1
  Assert10/1 -> X_valid/1
  DataReg_En3/1(Dout) -> ST8/1(In), Register13/1
  DataReg_En3/2(Valid) -> pulse_stretcher3/1(pulse_in)
  pulse_stretcher3/1(extd_out) -> Down Sample8/1
  Down Sample7/1 -> Assert11/1
  Register13/1 -> Down Sample7/1
  [CE_dest] -> pulse_stretcher3/2(clr)
  Convert/1 -> DataReg_En3/1(Din)
  Delay1/1 -> DataReg_En3/2(en)
  Assert11/1 -> Sum/1
  Assert12/1 -> Sum_valid/1
  Down Sample8/1 -> Assert12/1
  fifo_fofb_y/2(wr_full) -> Terminator7/1  "wr_full"

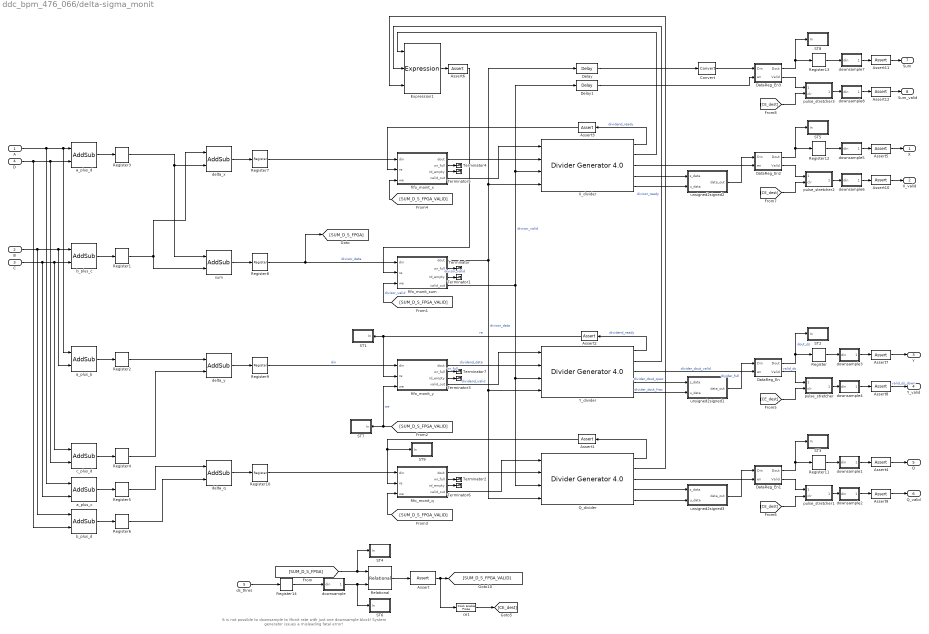
== system ddc_bpm_476_066/delta-sigma_monit ==
  note: It is not possible to downsample
      | to Monit rate with just one downsample block!
      | System generator issues a misleading fatal error!
  A : Inport
  B : Inport  Port=2
  C : Inport  Port=3
  D : Inport  Port=4
  ds_thres : Inport  Port=5
  Assert{,4..5,7..12} (9 alike) : xbsIndex_r4/Assert  assert_type=off  type_source=Explicitly  gui_display_data_type=Fixed-point  arith_type="Signed  (2's comp)"  n_bits=16  bin_pt=14  preci_type=Single  exp_width=8  frac_width=24  assert_rate=on  rate_source=Explicitly  period=(1/Fs_adc/n_ovs)*(R_fofb*R_sec*R_sec_cfir*R_sec_pfir*n_ovs)  output_port=on  block_type=assert
  Assert{1..3,6} (4 alike) : xbsIndex_r4/Assert  assert_type=off  type_source=Explicitly  gui_display_data_type=Fixed-point  arith_type="Signed  (2's comp)"  n_bits=16  bin_pt=14  preci_type=Single  exp_width=8  frac_width=24  assert_rate=on  rate_source=Explicitly  period=1/Fs_adc/n_ovs  output_port=on  block_type=assert
  Convert : xbsIndex_r4/Convert  gui_display_data_type=Fixed-point  arith_type="Signed  (2's comp)"  n_bits=25  bin_pt=21  float_type=Single  exp_bits=8  fraction_bits=24  quantization="Round  (unbiased: +/- Inf)"  overflow=Saturate  en=off  latency=0  dbl_ovrd=off  pipeline=off  block_type=convert
  DataReg_En : Subsystem
  DataReg_En1 : Subsystem
  DataReg_En2 : Subsystem
  DataReg_En3 : Subsystem
  Delay : xbsIndex_r4/Delay  rst=off  infoeditControl=Selection of Reset will increase slice count due to use of real FFs and instead of SRLs  en=off  latency=25  dbl_ovrd=off  reg_retiming=off  block_type=delay
  Delay1 : xbsIndex_r4/Delay  rst=off  infoeditControl=Selection of Reset will increase slice count due to use of real FFs and instead of SRLs  en=off  latency=25  dbl_ovrd=off  reg_retiming=off  block_type=delay
  Expression1 : xbsIndex_r4/Expression  expression=a & b & c  align_bp=on  en=off  latency=0  precision=Full  arith_type=Unsigned  n_bits=16  bin_pt=0  dbl_ovrd=off  block_type=expr
  Q_divider : xbsIndex_r4/Divider Generator 4.0   algorithm_type=High_Radix  remainder_type=Fractional  fractional_width=24  clocks_per_division=1  divide_by_zero_detect=off  flowcontrol=NonBlocking  optimizegoal=Performance  latency_configuration=Manual  latency=25  dividend_has_tuser=off  dividend_has_tlast=off  divisor_has_tuser=off  divisor_has_tlast=off  aclken=off  aresetn=off  outtready=off  outtlastbehv=Null  trim_axipin_name=on  dividend_tuser_width=1  divisor_tuser_width=1  operand_sign=Signed  dividend_and_quotient_width=16  divisor_width=16  ip_name=Divider Generator  ip_version=4.0  dsptool_ready=true  ipcore_usecache=true  ipcore_useipmodelcache=true  wrapper_available=true  port_translation_map={'aclken' => 'en','aresetn' => 'rst'}  ipcore_fpga_part=xlipgetpartsetting(gcb, {'virtex7', 'xc7v1500t', '-2', 'fhg1157'})  ipcore_verbose=false  block_type=div_gen_v4_0
      settings: infoedit=Divider Generator 4.0
  Register{,1..14} (15 alike) : xbsIndex_r4/Register  init=0  rst=off  en=off  dbl_ovrd=off  block_type=register
  Relational : xbsIndex_r4/Relational  mode=a>b  en=off  latency=1  dbl_ovrd=off  block_type=relational
  ST1 : Subsystem
  ST2 : Subsystem
  ST3 : Subsystem
  ST4 : Subsystem
  ST5 : Subsystem
  ST6 : Subsystem
  ST7 : Subsystem
  ST8 : Subsystem
  ST9 : Subsystem
  Terminator{,1..7} (8 alike) : Terminator
  X_divider : xbsIndex_r4/Divider Generator 4.0   algorithm_type=High_Radix  remainder_type=Fractional  fractional_width=24  clocks_per_division=1  divide_by_zero_detect=off  flowcontrol=NonBlocking  optimizegoal=Performance  latency_configuration=Manual  latency=25  dividend_has_tuser=off  dividend_has_tlast=off  divisor_has_tuser=off  divisor_has_tlast=off  aclken=off  aresetn=off  outtready=off  outtlastbehv=Null  trim_axipin_name=on  dividend_tuser_width=1  divisor_tuser_width=1  operand_sign=Signed  dividend_and_quotient_width=16  divisor_width=16  ip_name=Divider Generator  ip_version=4.0  dsptool_ready=true  ipcore_usecache=true  ipcore_useipmodelcache=true  wrapper_available=true  port_translation_map={'aclken' => 'en','aresetn' => 'rst'}  ipcore_fpga_part=xlipgetpartsetting(gcb, {'virtex7', 'xc7v1500t', '-2', 'fhg1157'})  ipcore_verbose=false  block_type=div_gen_v4_0
      settings: infoedit=Divider Generator 4.0
  Y_divider : xbsIndex_r4/Divider Generator 4.0   algorithm_type=High_Radix  remainder_type=Fractional  fractional_width=24  clocks_per_division=1  divide_by_zero_detect=off  flowcontrol=NonBlocking  optimizegoal=Performance  latency_configuration=Manual  latency=25  dividend_has_tuser=off  dividend_has_tlast=off  divisor_has_tuser=off  divisor_has_tlast=off  aclken=off  aresetn=off  outtready=off  outtlastbehv=Null  trim_axipin_name=on  dividend_tuser_width=1  divisor_tuser_width=1  operand_sign=Signed  dividend_and_quotient_width=16  divisor_width=16  ip_name=Divider Generator  ip_version=4.0  dsptool_ready=true  ipcore_usecache=true  ipcore_useipmodelcache=true  wrapper_available=true  port_translation_map={'aclken' => 'en','aresetn' => 'rst'}  ipcore_fpga_part=xlipgetpartsetting(gcb, {'virtex7', 'xc7v1500t', '-2', 'fhg1157'})  ipcore_verbose=false  block_type=div_gen_v4_0
      settings: infoedit=Divider Generator 4.0
  a_plus_b : xbsIndex_r4/AddSub  mode=Addition  use_carryin=off  use_carryout=off  en=off  latency=0  precision=Full  arith_type=Unsigned  n_bits=16  bin_pt=14  quantization=Truncate  overflow=Wrap  dbl_ovrd=off  use_behavioral_HDL=off  hw_selection=Fabric  pipelined=off  block_type=addsub
  a_plus_c : xbsIndex_r4/AddSub  mode=Addition  use_carryin=off  use_carryout=off  en=off  latency=0  precision=Full  arith_type=Unsigned  n_bits=16  bin_pt=14  quantization=Truncate  overflow=Wrap  dbl_ovrd=off  use_behavioral_HDL=off  hw_selection=Fabric  pipelined=off  block_type=addsub
  a_plus_d : xbsIndex_r4/AddSub  mode=Addition  use_carryin=off  use_carryout=off  en=off  latency=0  precision=Full  arith_type=Unsigned  n_bits=16  bin_pt=14  quantization=Truncate  overflow=Wrap  dbl_ovrd=off  use_behavioral_HDL=off  hw_selection=Fabric  pipelined=off  block_type=addsub
  b_plus_c : xbsIndex_r4/AddSub  mode=Addition  use_carryin=off  use_carryout=off  en=off  latency=0  precision=Full  arith_type=Unsigned  n_bits=16  bin_pt=14  quantization=Truncate  overflow=Wrap  dbl_ovrd=off  use_behavioral_HDL=off  hw_selection=Fabric  pipelined=off  block_type=addsub
  b_plus_d : xbsIndex_r4/AddSub  mode=Addition  use_carryin=off  use_carryout=off  en=off  latency=0  precision=Full  arith_type=Unsigned  n_bits=16  bin_pt=14  quantization=Truncate  overflow=Wrap  dbl_ovrd=off  use_behavioral_HDL=off  hw_selection=Fabric  pipelined=off  block_type=addsub
  c_plus_d : xbsIndex_r4/AddSub  mode=Addition  use_carryin=off  use_carryout=off  en=off  latency=0  precision=Full  arith_type=Unsigned  n_bits=16  bin_pt=14  quantization=Truncate  overflow=Wrap  dbl_ovrd=off  use_behavioral_HDL=off  hw_selection=Fabric  pipelined=off  block_type=addsub
  ce1 : xbsIndex_r4/Clock Enable Probe  inherit_constraints=on  block_type=ceprobe
      settings: infoedit="Clock enable extractor.  Produces a Boolean output that mirrors the hardware clock enable associated with the input sample rate.<br><br>Hardware notes: in hardware this block costs nothing."
  delta_q : xbsIndex_r4/AddSub  mode=Subtraction  use_carryin=off  use_carryout=off  en=off  latency=0  precision=Full  arith_type=Unsigned  n_bits=16  bin_pt=14  quantization=Truncate  overflow=Wrap  dbl_ovrd=off  use_behavioral_HDL=off  hw_selection=Fabric  pipelined=off  block_type=addsub
  delta_x : xbsIndex_r4/AddSub  mode=Subtraction  use_carryin=off  use_carryout=off  en=off  latency=0  precision=Full  arith_type=Unsigned  n_bits=16  bin_pt=14  quantization=Truncate  overflow=Wrap  dbl_ovrd=off  use_behavioral_HDL=off  hw_selection=Fabric  pipelined=off  block_type=addsub
  delta_y : xbsIndex_r4/AddSub  mode=Subtraction  use_carryin=off  use_carryout=off  en=off  latency=0  precision=Full  arith_type=Unsigned  n_bits=16  bin_pt=14  quantization=Truncate  overflow=Wrap  dbl_ovrd=off  use_behavioral_HDL=off  hw_selection=Fabric  pipelined=off  block_type=addsub
  downsample : Subsystem
  downsample1 : Subsystem
  downsample2 : Subsystem
  downsample3 : Subsystem
  downsample4 : Subsystem
  downsample5 : Subsystem
  downsample6 : Subsystem
  downsample7 : Subsystem
  downsample8 : Subsystem
  fifo_monit_q : Subsystem
  fifo_monit_sum : Subsystem
  fifo_monit_x : Subsystem
  fifo_monit_y : Subsystem
  pulse_stretcher : Subsystem
  pulse_stretcher1 : Subsystem
  pulse_stretcher2 : Subsystem
  pulse_stretcher3 : Subsystem
  sum : xbsIndex_r4/AddSub  mode=Addition  use_carryin=off  use_carryout=off  en=off  latency=0  precision=Full  arith_type=Unsigned  n_bits=16  bin_pt=14  quantization=Truncate  overflow=Wrap  dbl_ovrd=off  use_behavioral_HDL=off  hw_selection=Fabric  pipelined=off  block_type=addsub
  unsigned2signed1 : Subsystem
  unsigned2signed2 : Subsystem
  unsigned2signed3 : Subsystem
  X : Outport
  X_valid : Outport  Port=2
  Y : Outport  Port=3
  Y_valid : Outport  Port=4
  Q : Outport  Port=5
  Q_valid : Outport  Port=6
  Sum : Outport  Port=7
  Sum_valid : Outport  Port=8
  wires:
  A/1 -> a_plus_d/1, a_plus_b/1, a_plus_c/1
  D/1 -> a_plus_d/2, c_plus_d/2, b_plus_d/2
  B/1 -> b_plus_c/1, a_plus_b/2, b_plus_d/1
  C/1 -> b_plus_c/2, c_plus_d/1, a_plus_c/2
  a_plus_d/1 -> Register3/1
  b_plus_c/1 -> Register1/1
  a_plus_b/1 -> Register2/1
  c_plus_d/1 -> Register4/1
  a_plus_c/1 -> Register5/1
  b_plus_d/1 -> Register6/1
  Register3/1 -> sum/1, delta_x/2
  Register1/1 -> sum/2, delta_x/1
  Register2/1 -> delta_y/1
  Register4/1 -> delta_y/2
  Register5/1 -> delta_q/1
  Register6/1 -> delta_q/2
  delta_q/1 -> Register10/1
  delta_x/1 -> Register7/1
  Register8/1 -> fifo_monit_sum/1(din), [SUM_D_S_FPGA]  "divisor_data"
  sum/1 -> Register8/1
  delta_y/1 -> Register9/1
  Delay/1 -> Convert/1
  Register7/1 -> fifo_monit_x/1(din)
  Y_divider/5 -> unsigned2signed1/2(u_data)  "divider_dout_frac"
  Y_divider/3 -> DataReg_En/2(en)  "divider_dout_valid"
  Register9/1 -> fifo_monit_y/1(din)  "din"
  Register10/1 -> fifo_monit_q/1(din)
  X_divider/2 -> Expression1/1
  Y_divider/2 -> Expression1/2  "divisor_ready"
  ds_thres/1 -> Register14/1
  [SUM_D_S_FPGA] -> Relational/1, ST4/1(In)
  Relational/1 -> Assert/1
  fifo_monit_x/1(dout) -> X_divider/2
  fifo_monit_q/1(dout) -> Q_divider/2
  Q_divider/2 -> Expression1/3
  Q_divider/1 -> Assert1/1
  fifo_monit_q/4(valid_out) -> Q_divider/1
  fifo_monit_x/4(valid_out) -> X_divider/1
  X_divider/5 -> unsigned2signed2/2(u_data)
  X_divider/4 -> unsigned2signed2/1(s_data)
  Y_divider/4 -> unsigned2signed1/1(s_data)  "divider_dout_quoc"
  unsigned2signed1/1(data_out) -> DataReg_En/1(Din)  "divider_full"
  Q_divider/5 -> unsigned2signed3/2(u_data)
  Q_divider/4 -> unsigned2signed3/1(s_data)
  Assert/1 -> [SUM_D_S_FPGA_VALID], ce1/1
  downsample/1(dout) -> ST6/1(In), Relational/2
  fifo_monit_y/1(dout) -> Y_divider/2  "dividend_data"
  [SUM_D_S_FPGA_VALID] -> ST7/1(In), fifo_monit_y/3(we)  "we"
  [SUM_D_S_FPGA_VALID] -> fifo_monit_sum/3(we)  "divisor_valid"
  Expression1/1 -> Assert6/1
  [SUM_D_S_FPGA_VALID] -> fifo_monit_x/3(we)
  [SUM_D_S_FPGA_VALID] -> fifo_monit_q/3(we)
  fifo_monit_y/4(valid_out) -> Y_divider/1  "dividend_valid"
  fifo_monit_sum/4(valid_out) -> Q_divider/3, Y_divider/3, X_divider/3, Delay1/1  "divisor_valid"
  fifo_monit_sum/2(wr_full) -> Terminator/1  "divisor_valid"
  fifo_monit_sum/3(rd_empty) -> Terminator1/1
  fifo_monit_x/2(wr_full) -> Terminator4/1
  fifo_monit_x/3(rd_empty) -> Terminator5/1
  fifo_monit_sum/1(dout) -> Q_divider/4, Y_divider/4, X_divider/4, Delay/1  "divisor_data"
  fifo_monit_q/2(wr_full) -> Terminator2/1
  fifo_monit_y/3(rd_empty) -> Terminator3/1
  Register14/1 -> downsample/1(din)
  DataReg_En/1(Dout) -> ST2/1(In), Register/1  "dout_ds"
  fifo_monit_q/3(rd_empty) -> Terminator6/1
  Assert8/1 -> Y_valid/1  "valid_ds_down"
  Assert7/1 -> Y/1
  Assert1/1 -> ST9/1(In), fifo_monit_q/2(re)
  Assert2/1 -> ST1/1(In), fifo_monit_y/2(re)  "re"
  Assert3/1 -> fifo_monit_x/2(re)
  Assert6/1 -> fifo_monit_sum/2(re)
  Y_divider/1 -> Assert2/1  "dividend_ready"
  X_divider/1 -> Assert3/1  "dividend_ready"
  DataReg_En/2(Valid) -> pulse_stretcher/1(pulse_in)  "valid_ds"
  pulse_stretcher/1(extd_out) -> downsample4/1(din)
  downsample3/1(dout) -> Assert7/1
  downsample4/1(dout) -> Assert8/1
  Register/1 -> downsample3/1(din)
  ce1/1 -> [CE_dest]
  [CE_dest] -> pulse_stretcher/2(clr)
  unsigned2signed3/1(data_out) -> DataReg_En1/1(Din)
  DataReg_En1/1(Dout) -> ST3/1(In), Register11/1
  Assert9/1 -> Q_valid/1
  Assert4/1 -> Q/1
  DataReg_En1/2(Valid) -> pulse_stretcher1/1(pulse_in)
  pulse_stretcher1/1(extd_out) -> downsample2/1(din)
  downsample1/1(dout) -> Assert4/1
  downsample2/1(dout) -> Assert9/1
  Register11/1 -> downsample1/1(din)
  [CE_dest] -> pulse_stretcher1/2(clr)
  Q_divider/3 -> DataReg_En1/2(en)
  unsigned2signed2/1(data_out) -> DataReg_En2/1(Din)
  DataReg_En2/1(Dout) -> ST5/1(In), Register12/1
  DataReg_En2/2(Valid) -> pulse_stretcher2/1(pulse_in)
  pulse_stretcher2/1(extd_out) -> downsample6/1(din)
  downsample5/1(dout) -> Assert5/1
  downsample6/1(dout) -> Assert10/1
  Register12/1 -> downsample5/1(din)
  [CE_dest] -> pulse_stretcher2/2(clr)
  X_divider/3 -> DataReg_En2/2(en)
  Assert5/1 -> X/1
  Assert10/1 -> X_valid/1
  DataReg_En3/1(Dout) -> ST8/1(In), Register13/1
  DataReg_En3/2(Valid) -> pulse_stretcher3/1(pulse_in)
  pulse_stretcher3/1(extd_out) -> downsample8/1(din)
  downsample7/1(dout) -> Assert11/1
  Register13/1 -> downsample7/1(din)
  [CE_dest] -> pulse_stretcher3/2(clr)
  Convert/1 -> DataReg_En3/1(Din)
  Delay1/1 -> DataReg_En3/2(en)
  Assert11/1 -> Sum/1
  Assert12/1 -> Sum_valid/1
  downsample8/1(dout) -> Assert12/1
  fifo_monit_y/2(wr_full) -> Terminator7/1  "wr_full"
